simulink model "Combustion_Chamber"  (R2025a)
settings: Solver=VariableStepAuto  StartTime=0.0  StopTime=10.0  RelTol=1e-3
settings Model: Creator=ramch  LastModifiedBy=ramch

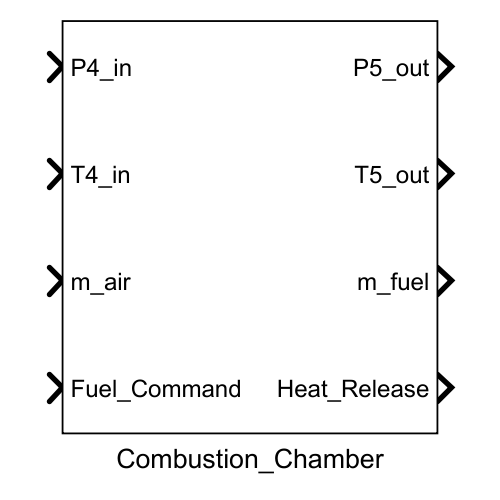
[thumbnail: Simulink's stored preview of the top-level diagram]
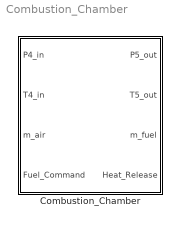
== system Combustion_Chamber ==
  Combustion_Chamber : Subsystem

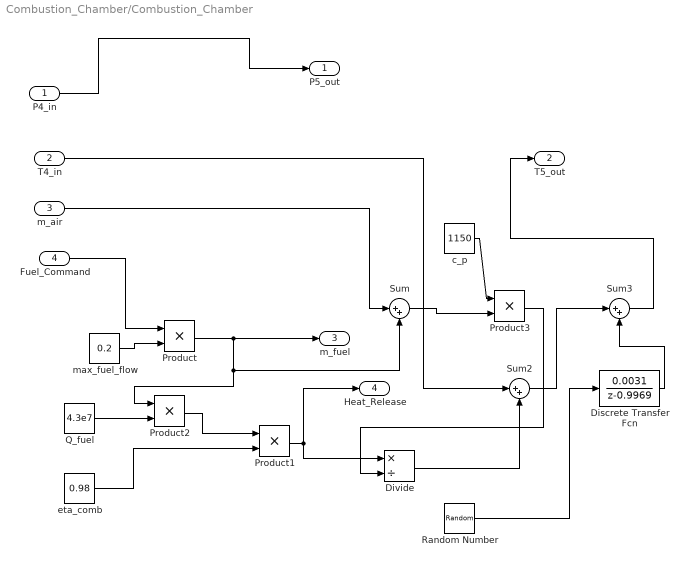
== system Combustion_Chamber/Combustion_Chamber ==
  P4_in : Inport
  T4_in : Inport  Port=2
  m_air : Inport  Port=3
  Fuel_Command : Inport  Port=4
  Discrete Transfer Fcn : DiscreteTransferFcn  Numerator=0.0031  Denominator=1 -0.9969  InitialStates=0.001
  Divide : Product  Inputs=*/
  Product{,1..3} (4 alike) : Product
  Q_fuel : Constant  Value=4.3e7
  Random Number : RandomNumber  Variance=0.5  SampleTime=0.001
  Sum : Sum  Inputs=|++
  Sum2 : Sum  Inputs=|++
  Sum3 : Sum  Inputs=|++
  c_p : Constant  Value=1150
  eta_comb : Constant  Value=0.98
  max_fuel_flow : Constant  Value=0.2
  P5_out : Outport
  T5_out : Outport  Port=2
  m_fuel : Outport  Port=3
  Heat_Release : Outport  Port=4
  wires:
  Fuel_Command/1 -> Product/1
  max_fuel_flow/1 -> Product/2
  Q_fuel/1 -> Product2/2
  eta_comb/1 -> Product1/2
  Product1/1 -> Heat_Release/1, Divide/1
  Product/1 -> Product2/1, Sum/2, m_fuel/1
  Product2/1 -> Product1/1
  m_air/1 -> Sum/1
  P4_in/1 -> P5_out/1
  Sum/1 -> Product3/2
  c_p/1 -> Product3/1
  Product3/1 -> Divide/2
  T4_in/1 -> Sum2/1
  Divide/1 -> Sum2/2
  Random Number/1 -> Discrete Transfer Fcn/1
  Sum3/1 -> T5_out/1
  Sum2/1 -> Sum3/1
  Discrete Transfer Fcn/1 -> Sum3/2
